simulink model "ThrottlePositionControlComposition"  (R2025a)
settings: Solver=FixedStepDiscrete  StartTime=0.0  StopTime=10.0  RelTol=1e-3  EnableMultiTasking=on
undefined symbols (not defined in the file or in its folder): D1, P
settings Model: Creator=z004f2se  LastModifiedBy=z004f2se
settings SolverCC: AutoInsertRateTranBlk=on
settings DataIOCC: SaveFormat=StructureWithTime
settings OptimizationCC: DefaultParameterBehavior=Inlined  EnhancedBackFolding=on  PassReuseOutputArgsAs=Individual arguments  ZeroExternalMemoryAtStartup=off  ZeroInternalMemoryAtStartup=off  OptimizeBlockOrder=speed  DifferentSizesBufferReuse=on  OptimizationCustomize=off  EfficientTunableParamExpr=on
settings DebuggingCC: ParameterTunabilityLossMsg=error
settings ModelReferenceCC: ModelReferenceNumInstancesAllowed=Single
settings SFSimCC: MATLABDynamicMemAlloc=off
settings RTWCC: SystemTargetFile=autosar.tlc  GenCodeOnly=on  TemplateMakefile=ert_default_tmf  DataTypeReplacement=CDataTypesFixedWidth  Description=AUTOSAR
settings CodeAppCC: ForceParamTrailComments=on  IgnoreCustomStorageClasses=off  OperatorAnnotations=on  SimulinkDataObjDesc=on  SFDataObjDesc=on  InsertBlockDesc=on
settings STFCustomTargetCC: SystemTargetFile=autosar.tlc  TargetLangStandard=C99 (ISO)  MultiwordLength=256.0  DynamicStringBufferSize=256.0  ParMdlRefBuildCompliant=on  CompOptLevelCompliant=on  IncludeMdlTerminateFcn=off  CombineOutputUpdateFcns=on  SuppressErrorStatus=on  ERTCustomFileBanners=on  SubcomponentCodeInterfacePackaging=Nonreusable function  SupportNonFinite=off  SupportComplex=off  SupportContinuousTime=off  SupportNonInlinedSFcns=off  RemoveResetFunc=on  MATLABClassNameForMDSCustomization=Simulink.SoftwareTarget.ERTCustomization  AutosarCompliant=on  GRTInterface=off  UseToolchainInfoCompliant=on  LookupTableObjectStructAxisOrder=2,1,3,4,...  LUTObjectStructOrderEvenSpacing=Size,Table,Breakpoints  AutosarCompilerAbstraction=off  AutosarMatrixIOAsArray=off  AutosarSchemaVersion=4.2  DisableAUTOSARRoutinesHostLibrary=off  AutosarMaxShortNameLength=128.0
settings ERTTargetCC: ExtModeTransport=0.0  ExtModeStaticAlloc=off  ExtModeMexFile=ext_comm  ExtModeIntrfLevel=Level1  ERTCustomFileTemplate=example_file_process.tlc  BooleanTrueId=TRUE  BooleanFalseId=FALSE  TargetLangStandard=C99 (ISO)  ConcurrentExecutionCompliant=off  IncludeMdlTerminateFcn=off  SuppressErrorStatus=on  SubcomponentCodeInterfacePackaging=Nonreusable function  SupportNonFinite=off  SupportComplex=off  ModelStepFunctionPrototypeControlCompliant=off  CPPClassGenCompliant=off  AutosarCompliant=on  LookupTableObjectStructAxisOrder=2,1,3,4,...  LUTObjectStructOrderEvenSpacing=Size,Table,Breakpoints

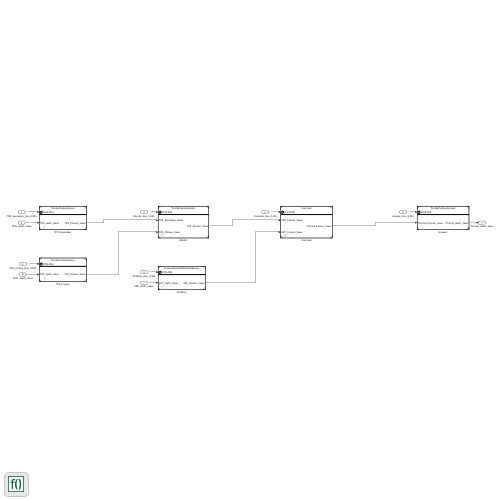
[thumbnail: Simulink's stored preview of the top-level diagram]
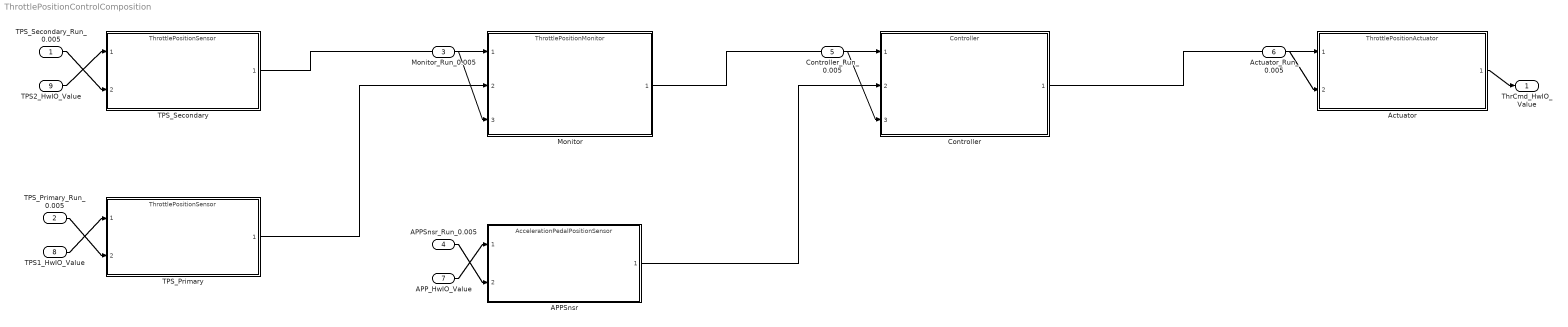
== system ThrottlePositionControlComposition ==
  TPS_Secondary_Run_0.005 : Inport  SampleTime=0.005  OutputFunctionCall=on
  TPS_Primary_Run_0.005 : Inport  Port=2  SampleTime=0.005  OutputFunctionCall=on
  Monitor_Run_0.005 : Inport  Port=3  SampleTime=0.005  OutputFunctionCall=on
  APPSnsr_Run_0.005 : Inport  Port=4  SampleTime=0.005  OutputFunctionCall=on
  Controller_Run_0.005 : Inport  Port=5  SampleTime=0.005  OutputFunctionCall=on
  Actuator_Run_0.005 : Inport  Port=6  SampleTime=0.005  OutputFunctionCall=on
  APP_HwIO_Value : Inport  Port=7  OutDataTypeStr=uint16  PortDimensions=1
  TPS1_HwIO_Value : Inport  Port=8  OutDataTypeStr=uint16  PortDimensions=1
  TPS2_HwIO_Value : Inport  Port=9  OutDataTypeStr=uint16  PortDimensions=1
  APPSnsr : ModelReference  ModelNameDialog=AccelerationPedalPositionSensor  SimulationMode=Normal  ScheduleRates=on  PortDiscreteRates=[0.005]  CachedPortDiscreteRates=[0.005]  ModelEventPortInfo=P:D1[0.005][0][0]  ModelReferenceVersion=1.1
  Actuator : ModelReference  ModelNameDialog=ThrottlePositionActuator  SimulationMode=Normal  ScheduleRates=on  PortDiscreteRates=[0.005]  CachedPortDiscreteRates=[0.005]  ModelEventPortInfo=P:D1[0.005][0][0]  ModelReferenceVersion=1.1
  Controller : ModelReference  ModelNameDialog=Controller  SimulationMode=Normal  ScheduleRates=on  PortDiscreteRates=[0.005]  CachedPortDiscreteRates=[0.005]  ModelEventPortInfo=P:D1[0.005][0][0]  ModelReferenceVersion=1.1
  Monitor : ModelReference  ModelNameDialog=ThrottlePositionMonitor  SimulationMode=Normal  ScheduleRates=on  PortDiscreteRates=[0.005]  CachedPortDiscreteRates=[0.005]  ModelEventPortInfo=P:D1[0.005][0][0]  ModelReferenceVersion=1.1
  TPS_Primary : ModelReference  ModelNameDialog=ThrottlePositionSensor  SimulationMode=Normal  ScheduleRates=on  PortDiscreteRates=[0.005]  CachedPortDiscreteRates=[0.005]  ModelEventPortInfo=P:D1[0.005][0][0]  ModelReferenceVersion=1.1
  TPS_Secondary : ModelReference  ModelNameDialog=ThrottlePositionSensor  SimulationMode=Normal  ScheduleRates=on  PortDiscreteRates=[0.005]  CachedPortDiscreteRates=[0.005]  ModelEventPortInfo=P:D1[0.005][0][0]  ModelReferenceVersion=1.1
  ThrCmd_HwIO_Value : Outport  OutDataTypeStr=int16  PortDimensions=1
  wires:
  TPS_Secondary_Run_0.005/1 -> TPS_Secondary/2
  TPS_Primary_Run_0.005/1 -> TPS_Primary/2
  Monitor_Run_0.005/1 -> Monitor/3
  APPSnsr_Run_0.005/1 -> APPSnsr/2
  Controller_Run_0.005/1 -> Controller/3
  Actuator_Run_0.005/1 -> Actuator/2
  APPSnsr/1 -> Controller/2
  Controller/1 -> Actuator/1
  Monitor/1 -> Controller/1
  TPS_Primary/1 -> Monitor/2
  TPS_Secondary/1 -> Monitor/1
  APP_HwIO_Value/1 -> APPSnsr/1
  Actuator/1 -> ThrCmd_HwIO_Value/1
  TPS1_HwIO_Value/1 -> TPS_Primary/1
  TPS2_HwIO_Value/1 -> TPS_Secondary/1
